simulink model "ctrl_student_HIL_Modules_withoutPathParam"  (R2015a)
settings: Solver=ode3  SolverMode=SingleTasking  StartTime=0.0  StopTime=inf  FixedStep=0.01  RelTol=1e-3
values from neighbouring files (symbols this model uses):
  D = [d_11 d_12 0 ... (first row only)    [ctrl_student_init.m]    (also in ctrl_student_observer_D.m = reshape([u.*(-3.545e-1)+u.^2.*3.787+6.555e-1,0.0,0.0,v.*2.44)
  eta_dot_ini = [7;0;0]    [Innput.m]    (also in Input_v3.m)
  K2 = diag([200,50,3])    [Input_v3.m]    (also in inputDPgains.m = [1 0 0; 0 1 0; 0 0 1])
  K_SZ = [1;1]    [Innput.m]
  l1 = [1 0 0;0 1 0;0 0 0.05]    [Input_v3.m]    (also in inputDPgains.m = [1 0 0; 0 1 0; 0 0 1])
  l2 = [1 0 0;0 1 0;0 0 0.05]    [Input_v3.m]    (also in inputDPgains.m = [1 0 0; 0 1 0; 0 0 1])
  l3 = [1 0 0;0 1 0;0 0 0.05]    [Input_v3.m]    (also in inputDPgains.m = [1 0 0; 0 1 0; 0 0 1])
  lim = [1.00;-20;6.45/2;-6.45/2]    [Innput.m]    (also in Input_v3.m = [20;-20;9;-9])
  lim_2 = [1.5;-22;7;-7]    [Innput.m]    (also in Input_v3.m = [25;-25;10;-10])
  M = [m_11 0    0 ... (first row only)    [ctrl_student_init.m]
libraries: dspstat3 x1, simulink x1
(part 1 of 3)
settings Model: CovSFcnEnable=off  Creator=mclab  LastModifiedBy=MCLab
settings OptimizationCC: BlockReduction=off  BooleanDataType=off
settings DebuggingCC: SaveWithParameterizedLinksMsg=none  UnderspecifiedInitializationDetection=Classic  MergeDetectMultiDrivingBlocksExec=none  SignalResolutionControl=TryResolveAllWithWarning
settings HardwareCC: TargetLongLongMode=on  TargetIntDivRoundTo=Zero  TargetEndianess=LittleEndian  TargetHWDeviceType=MATLAB Host  ProdEqTarget=off

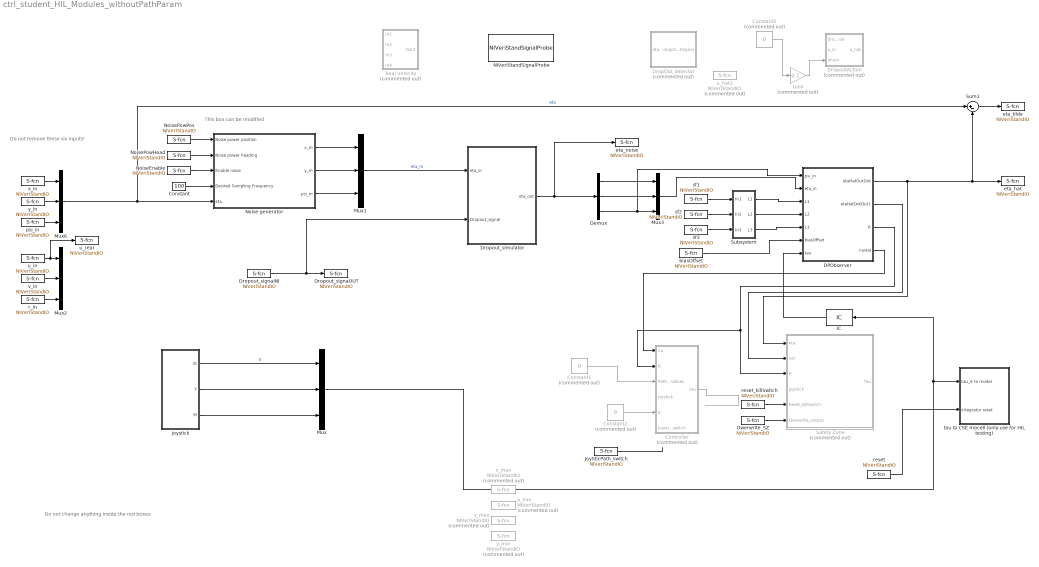
== system ctrl_student_HIL_Modules_withoutPathParam ==
  note: This box can be modified
  note: Do not change anything inside the red boxes
  note: Do not remove these six inputs!
  Constant : Constant  Value=100
  Constant1 : Constant  Commented=on  Value=0
  Constant2 : Constant  Commented=on  Value=0
  Constant5 : Constant  Commented=on  Value=0
  Controller : Subsystem  Commented=on
  DPObserver : Subsystem
  Demux : Demux  Outputs=3
  DropOut_detector : Subsystem  Commented=on
  DropoutAction : Subsystem  Commented=on
  Dropout_signaINl : S-Function  Priority=15  FunctionName=NIVeriStandIO  Parameters=width dtype portnum stime stype btype  mask(NI VeriStand Inport){portnum=15, width=-1, stime=-1, dtype=auto, stype=auto, btype=1}
      mask prompts: portnum "Port number:"; width "Port dimensions (-1 for dynamically sized):"; stime "Sample time (-1 for inherited):"; dtype "Data type:"; stype "Signal type:"; btype "Block type:"
      mask help: Use this inport on any level of nested subsystems to allow NI VeriStand software to map signals to it.
      mask init:
      | NIVeriStandIO_init;
      settings: CopyFcn=NIVeriStand_MDL_functions('', 'IO_copy');  DeleteFcn=NIVeriStand_MDL_functions('', 'IO_delete');  MoveFcn=set_param(gcb, 'Mask', 'on');
      mask Callback portnum: NIVeriStand_MDL_functions('', 'IO_setportnum');
      mask TypeOptions dtype: auto | double | single | int8 | uint8 | int16 | uint16 | int32 | uint32 | boolean
      mask Callback dtype: NIVeriStand_MDL_functions('', 'IO_booleansignal');
      mask TypeOptions stype: auto | real | complex
      mask Display:
      | patch([-x x], [-y y], [.90980 .81960 .32156]);
      | plot([xrad -x x xrad], [yrad -y y yrad]);
      | fprintf('NI In%d', portnum);
  Dropout_signaOUT : S-Function  Priority=5  FunctionName=NIVeriStandIO  Parameters=width dtype portnum stime stype btype  mask(NI VeriStand Outport){portnum=5, width=-1, stime=-1, dtype=auto, stype=auto, btype=0}
      mask prompts: portnum "Port number:"; width "Port dimensions (-1 for dynamically sized):"; stime "Sample time (-1 for inherited):"; dtype "Data type:"; stype "Signal type:"; btype "Block type:"
      mask help: Use this outport on any level of nested subsystems to allow NI VeriStand software to map signals to it.
      mask init:
      | NIVeriStandIO_init;
      settings: CopyFcn=NIVeriStand_MDL_functions('', 'IO_copy');  DeleteFcn=NIVeriStand_MDL_functions('', 'IO_delete');  MoveFcn=set_param(gcb, 'Mask', 'on');
      mask Callback portnum: NIVeriStand_MDL_functions('', 'IO_setportnum');
      mask TypeOptions dtype: auto | double | single | int8 | uint8 | int16 | uint16 | int32 | uint32 | boolean
      mask Callback dtype: NIVeriStand_MDL_functions('', 'IO_booleansignal');
      mask TypeOptions stype: auto | real | complex
      mask Display:
      | patch([-x x], [-y y], [.90980 .81960 .32156]);
      | plot([xrad -x x xrad], [yrad -y y yrad]);
      | fprintf('NI Out%d', portnum);
  Dropout_simulator : Subsystem
  Gain : Gain  Commented=on  Gain=0.1
  IC : InitialCondition  Value=[0;0;0]
  JoySticPath_switch : S-Function  Priority=16  FunctionName=NIVeriStandIO  Parameters=width dtype portnum stime stype btype  mask(NI VeriStand Inport){portnum=16, width=-1, stime=-1, dtype=auto, stype=auto, btype=1}
      mask prompts: portnum "Port number:"; width "Port dimensions (-1 for dynamically sized):"; stime "Sample time (-1 for inherited):"; dtype "Data type:"; stype "Signal type:"; btype "Block type:"
      mask help: Use this inport on any level of nested subsystems to allow NI VeriStand software to map signals to it.
      mask init:
      | NIVeriStandIO_init;
      settings: CopyFcn=NIVeriStand_MDL_functions('', 'IO_copy');  DeleteFcn=NIVeriStand_MDL_functions('', 'IO_delete');  MoveFcn=set_param(gcb, 'Mask', 'on');
      mask Callback portnum: NIVeriStand_MDL_functions('', 'IO_setportnum');
      mask TypeOptions dtype: auto | double | single | int8 | uint8 | int16 | uint16 | int32 | uint32 | boolean
      mask Callback dtype: NIVeriStand_MDL_functions('', 'IO_booleansignal');
      mask TypeOptions stype: auto | real | complex
      mask Display:
      | patch([-x x], [-y y], [.90980 .81960 .32156]);
      | plot([xrad -x x xrad], [yrad -y y yrad]);
      | fprintf('NI In%d', portnum);
  Mux{,1..3,6} (5 alike) : Mux  Inputs=3
  NIVeriStandSignalProbe : S-Function  FunctionName=NIVeriStandSignalProbe  Parameters=1
  Noise generator : Subsystem
  NoiseEnable : S-Function  Priority=5  FunctionName=NIVeriStandIO  Parameters=width dtype portnum stime stype btype  mask(NI VeriStand Inport){portnum=5, width=-1, stime=-1, dtype=auto, stype=auto, btype=1}
      mask prompts: portnum "Port number:"; width "Port dimensions (-1 for dynamically sized):"; stime "Sample time (-1 for inherited):"; dtype "Data type:"; stype "Signal type:"; btype "Block type:"
      mask help: Use this inport on any level of nested subsystems to allow NI VeriStand software to map signals to it.
      mask init:
      | NIVeriStandIO_init;
      settings: CopyFcn=NIVeriStand_MDL_functions('', 'IO_copy');  DeleteFcn=NIVeriStand_MDL_functions('', 'IO_delete');  MoveFcn=set_param(gcb, 'Mask', 'on');
      mask Callback portnum: NIVeriStand_MDL_functions('', 'IO_setportnum');
      mask TypeOptions dtype: auto | double | single | int8 | uint8 | int16 | uint16 | int32 | uint32 | boolean
      mask Callback dtype: NIVeriStand_MDL_functions('', 'IO_booleansignal');
      mask TypeOptions stype: auto | real | complex
      mask Display:
      | patch([-x x], [-y y], [.90980 .81960 .32156]);
      | plot([xrad -x x xrad], [yrad -y y yrad]);
      | fprintf('NI In%d', portnum);
  NoisePowHead : S-Function  Priority=6  FunctionName=NIVeriStandIO  Parameters=width dtype portnum stime stype btype  mask(NI VeriStand Inport){portnum=6, width=-1, stime=-1, dtype=auto, stype=auto, btype=1}
      mask prompts: portnum "Port number:"; width "Port dimensions (-1 for dynamically sized):"; stime "Sample time (-1 for inherited):"; dtype "Data type:"; stype "Signal type:"; btype "Block type:"
      mask help: Use this inport on any level of nested subsystems to allow NI VeriStand software to map signals to it.
      mask init:
      | NIVeriStandIO_init;
      settings: CopyFcn=NIVeriStand_MDL_functions('', 'IO_copy');  DeleteFcn=NIVeriStand_MDL_functions('', 'IO_delete');  MoveFcn=set_param(gcb, 'Mask', 'on');
      mask Callback portnum: NIVeriStand_MDL_functions('', 'IO_setportnum');
      mask TypeOptions dtype: auto | double | single | int8 | uint8 | int16 | uint16 | int32 | uint32 | boolean
      mask Callback dtype: NIVeriStand_MDL_functions('', 'IO_booleansignal');
      mask TypeOptions stype: auto | real | complex
      mask Display:
      | patch([-x x], [-y y], [.90980 .81960 .32156]);
      | plot([xrad -x x xrad], [yrad -y y yrad]);
      | fprintf('NI In%d', portnum);
  NoisePowPos : S-Function  Priority=9  FunctionName=NIVeriStandIO  Parameters=width dtype portnum stime stype btype  mask(NI VeriStand Inport){portnum=9, width=-1, stime=-1, dtype=auto, stype=auto, btype=1}
      mask prompts: portnum "Port number:"; width "Port dimensions (-1 for dynamically sized):"; stime "Sample time (-1 for inherited):"; dtype "Data type:"; stype "Signal type:"; btype "Block type:"
      mask help: Use this inport on any level of nested subsystems to allow NI VeriStand software to map signals to it.
      mask init:
      | NIVeriStandIO_init;
      settings: CopyFcn=NIVeriStand_MDL_functions('', 'IO_copy');  DeleteFcn=NIVeriStand_MDL_functions('', 'IO_delete');  MoveFcn=set_param(gcb, 'Mask', 'on');
      mask Callback portnum: NIVeriStand_MDL_functions('', 'IO_setportnum');
      mask TypeOptions dtype: auto | double | single | int8 | uint8 | int16 | uint16 | int32 | uint32 | boolean
      mask Callback dtype: NIVeriStand_MDL_functions('', 'IO_booleansignal');
      mask TypeOptions stype: auto | real | complex
      mask Display:
      | patch([-x x], [-y y], [.90980 .81960 .32156]);
      | plot([xrad -x x xrad], [yrad -y y yrad]);
      | fprintf('NI In%d', portnum);
  Owerwrite_SZ : S-Function  Priority=18  FunctionName=NIVeriStandIO  Parameters=width dtype portnum stime stype btype  mask(NI VeriStand Inport){portnum=18, width=-1, stime=-1, dtype=auto, stype=auto, btype=1}
      mask prompts: portnum "Port number:"; width "Port dimensions (-1 for dynamically sized):"; stime "Sample time (-1 for inherited):"; dtype "Data type:"; stype "Signal type:"; btype "Block type:"
      mask help: Use this inport on any level of nested subsystems to allow NI VeriStand software to map signals to it.
      mask init:
      | NIVeriStandIO_init;
      settings: CopyFcn=NIVeriStand_MDL_functions('', 'IO_copy');  DeleteFcn=NIVeriStand_MDL_functions('', 'IO_delete');  MoveFcn=set_param(gcb, 'Mask', 'on');
      mask Callback portnum: NIVeriStand_MDL_functions('', 'IO_setportnum');
      mask TypeOptions dtype: auto | double | single | int8 | uint8 | int16 | uint16 | int32 | uint32 | boolean
      mask Callback dtype: NIVeriStand_MDL_functions('', 'IO_booleansignal');
      mask TypeOptions stype: auto | real | complex
      mask Display:
      | patch([-x x], [-y y], [.90980 .81960 .32156]);
      | plot([xrad -x x xrad], [yrad -y y yrad]);
      | fprintf('NI In%d', portnum);
  Real Velocity : Subsystem  Commented=on
  "Safety Zone " : Subsystem  Commented=on
  Subsystem : Subsystem
  Sum1 : Sum  Inputs=|+-
  biasOffset : S-Function  Priority=13  FunctionName=NIVeriStandIO  Parameters=width dtype portnum stime stype btype  mask(NI VeriStand Inport){portnum=13, width=-1, stime=-1, dtype=auto, stype=auto, btype=1}
      mask prompts: portnum "Port number:"; width "Port dimensions (-1 for dynamically sized):"; stime "Sample time (-1 for inherited):"; dtype "Data type:"; stype "Signal type:"; btype "Block type:"
      mask help: Use this inport on any level of nested subsystems to allow NI VeriStand software to map signals to it.
      mask init:
      | NIVeriStandIO_init;
      settings: CopyFcn=NIVeriStand_MDL_functions('', 'IO_copy');  DeleteFcn=NIVeriStand_MDL_functions('', 'IO_delete');  MoveFcn=set_param(gcb, 'Mask', 'on');
      mask Callback portnum: NIVeriStand_MDL_functions('', 'IO_setportnum');
      mask TypeOptions dtype: auto | double | single | int8 | uint8 | int16 | uint16 | int32 | uint32 | boolean
      mask Callback dtype: NIVeriStand_MDL_functions('', 'IO_booleansignal');
      mask TypeOptions stype: auto | real | complex
      mask Display:
      | patch([-x x], [-y y], [.90980 .81960 .32156]);
      | plot([xrad -x x xrad], [yrad -y y yrad]);
      | fprintf('NI In%d', portnum);
  eta_hat : S-Function  Priority=1  FunctionName=NIVeriStandIO  Parameters=width dtype portnum stime stype btype  mask(NI VeriStand Outport){portnum=1, width=-1, stime=-1, dtype=auto, stype=auto, btype=0}
      mask prompts: portnum "Port number:"; width "Port dimensions (-1 for dynamically sized):"; stime "Sample time (-1 for inherited):"; dtype "Data type:"; stype "Signal type:"; btype "Block type:"
      mask help: Use this outport on any level of nested subsystems to allow NI VeriStand software to map signals to it.
      mask init:
      | NIVeriStandIO_init;
      settings: CopyFcn=NIVeriStand_MDL_functions('', 'IO_copy');  DeleteFcn=NIVeriStand_MDL_functions('', 'IO_delete');  MoveFcn=set_param(gcb, 'Mask', 'on');
      mask Callback portnum: NIVeriStand_MDL_functions('', 'IO_setportnum');
      mask TypeOptions dtype: auto | double | single | int8 | uint8 | int16 | uint16 | int32 | uint32 | boolean
      mask Callback dtype: NIVeriStand_MDL_functions('', 'IO_booleansignal');
      mask TypeOptions stype: auto | real | complex
      mask Display:
      | patch([-x x], [-y y], [.90980 .81960 .32156]);
      | plot([xrad -x x xrad], [yrad -y y yrad]);
      | fprintf('NI Out%d', portnum);
  eta_noise : S-Function  Priority=4  FunctionName=NIVeriStandIO  Parameters=width dtype portnum stime stype btype  mask(NI VeriStand Outport){portnum=4, width=-1, stime=-1, dtype=auto, stype=auto, btype=0}
      mask prompts: portnum "Port number:"; width "Port dimensions (-1 for dynamically sized):"; stime "Sample time (-1 for inherited):"; dtype "Data type:"; stype "Signal type:"; btype "Block type:"
      mask help: Use this outport on any level of nested subsystems to allow NI VeriStand software to map signals to it.
      mask init:
      | NIVeriStandIO_init;
      settings: CopyFcn=NIVeriStand_MDL_functions('', 'IO_copy');  DeleteFcn=NIVeriStand_MDL_functions('', 'IO_delete');  MoveFcn=set_param(gcb, 'Mask', 'on');
      mask Callback portnum: NIVeriStand_MDL_functions('', 'IO_setportnum');
      mask TypeOptions dtype: auto | double | single | int8 | uint8 | int16 | uint16 | int32 | uint32 | boolean
      mask Callback dtype: NIVeriStand_MDL_functions('', 'IO_booleansignal');
      mask TypeOptions stype: auto | real | complex
      mask Display:
      | patch([-x x], [-y y], [.90980 .81960 .32156]);
      | plot([xrad -x x xrad], [yrad -y y yrad]);
      | fprintf('NI Out%d', portnum);
  eta_tilde : S-Function  Priority=3  FunctionName=NIVeriStandIO  Parameters=width dtype portnum stime stype btype  mask(NI VeriStand Outport){portnum=3, width=-1, stime=-1, dtype=auto, stype=auto, btype=0}
      mask prompts: portnum "Port number:"; width "Port dimensions (-1 for dynamically sized):"; stime "Sample time (-1 for inherited):"; dtype "Data type:"; stype "Signal type:"; btype "Block type:"
      mask help: Use this outport on any level of nested subsystems to allow NI VeriStand software to map signals to it.
      mask init:
      | NIVeriStandIO_init;
      settings: CopyFcn=NIVeriStand_MDL_functions('', 'IO_copy');  DeleteFcn=NIVeriStand_MDL_functions('', 'IO_delete');  MoveFcn=set_param(gcb, 'Mask', 'on');
      mask Callback portnum: NIVeriStand_MDL_functions('', 'IO_setportnum');
      mask TypeOptions dtype: auto | double | single | int8 | uint8 | int16 | uint16 | int32 | uint32 | boolean
      mask Callback dtype: NIVeriStand_MDL_functions('', 'IO_booleansignal');
      mask TypeOptions stype: auto | real | complex
      mask Display:
      | patch([-x x], [-y y], [.90980 .81960 .32156]);
      | plot([xrad -x x xrad], [yrad -y y yrad]);
      | fprintf('NI Out%d', portnum);
  joystick : Subsystem
  psi_in : S-Function  Priority=2  FunctionName=NIVeriStandIO  Parameters=width dtype portnum stime stype btype  mask(NI VeriStand Inport){portnum=2, width=-1, stime=-1, dtype=auto, stype=auto, btype=1}
      mask prompts: portnum "Port number:"; width "Port dimensions (-1 for dynamically sized):"; stime "Sample time (-1 for inherited):"; dtype "Data type:"; stype "Signal type:"; btype "Block type:"
      mask help: Use this inport on any level of nested subsystems to allow NI VeriStand software to map signals to it.
      mask init:
      | NIVeriStandIO_init;
      settings: CopyFcn=NIVeriStand_MDL_functions('', 'IO_copy');  DeleteFcn=NIVeriStand_MDL_functions('', 'IO_delete');  MoveFcn=set_param(gcb, 'Mask', 'on');
      mask Callback portnum: NIVeriStand_MDL_functions('', 'IO_setportnum');
      mask TypeOptions dtype: auto | double | single | int8 | uint8 | int16 | uint16 | int32 | uint32 | boolean
      mask Callback dtype: NIVeriStand_MDL_functions('', 'IO_booleansignal');
      mask TypeOptions stype: auto | real | complex
      mask Display:
      | patch([-x x], [-y y], [.90980 .81960 .32156]);
      | plot([xrad -x x xrad], [yrad -y y yrad]);
      | fprintf('NI In%d', portnum);
  r_in : S-Function  Priority=4  FunctionName=NIVeriStandIO  Parameters=width dtype portnum stime stype btype  mask(NI VeriStand Inport){portnum=4, width=-1, stime=-1, dtype=auto, stype=auto, btype=1}
      mask prompts: portnum "Port number:"; width "Port dimensions (-1 for dynamically sized):"; stime "Sample time (-1 for inherited):"; dtype "Data type:"; stype "Signal type:"; btype "Block type:"
      mask help: Use this inport on any level of nested subsystems to allow NI VeriStand software to map signals to it.
      mask init:
      | NIVeriStandIO_init;
      settings: CopyFcn=NIVeriStand_MDL_functions('', 'IO_copy');  DeleteFcn=NIVeriStand_MDL_functions('', 'IO_delete');  MoveFcn=set_param(gcb, 'Mask', 'on');
      mask Callback portnum: NIVeriStand_MDL_functions('', 'IO_setportnum');
      mask TypeOptions dtype: auto | double | single | int8 | uint8 | int16 | uint16 | int32 | uint32 | boolean
      mask Callback dtype: NIVeriStand_MDL_functions('', 'IO_booleansignal');
      mask TypeOptions stype: auto | real | complex
      mask Display:
      | patch([-x x], [-y y], [.90980 .81960 .32156]);
      | plot([xrad -x x xrad], [yrad -y y yrad]);
      | fprintf('NI In%d', portnum);
  reset : S-Function  Priority=14  FunctionName=NIVeriStandIO  Parameters=width dtype portnum stime stype btype  mask(NI VeriStand Inport){portnum=14, width=-1, stime=-1, dtype=auto, stype=auto, btype=1}
      mask prompts: portnum "Port number:"; width "Port dimensions (-1 for dynamically sized):"; stime "Sample time (-1 for inherited):"; dtype "Data type:"; stype "Signal type:"; btype "Block type:"
      mask help: Use this inport on any level of nested subsystems to allow NI VeriStand software to map signals to it.
      mask init:
      | NIVeriStandIO_init;
      settings: CopyFcn=NIVeriStand_MDL_functions('', 'IO_copy');  DeleteFcn=NIVeriStand_MDL_functions('', 'IO_delete');  MoveFcn=set_param(gcb, 'Mask', 'on');
      mask Callback portnum: NIVeriStand_MDL_functions('', 'IO_setportnum');
      mask TypeOptions dtype: auto | double | single | int8 | uint8 | int16 | uint16 | int32 | uint32 | boolean
      mask Callback dtype: NIVeriStand_MDL_functions('', 'IO_booleansignal');
      mask TypeOptions stype: auto | real | complex
      mask Display:
      | patch([-x x], [-y y], [.90980 .81960 .32156]);
      | plot([xrad -x x xrad], [yrad -y y yrad]);
      | fprintf('NI In%d', portnum);
  reset_killSwitch : S-Function  Priority=17  FunctionName=NIVeriStandIO  Parameters=width dtype portnum stime stype btype  mask(NI VeriStand Inport){portnum=17, width=-1, stime=-1, dtype=auto, stype=auto, btype=1}
      mask prompts: portnum "Port number:"; width "Port dimensions (-1 for dynamically sized):"; stime "Sample time (-1 for inherited):"; dtype "Data type:"; stype "Signal type:"; btype "Block type:"
      mask help: Use this inport on any level of nested subsystems to allow NI VeriStand software to map signals to it.
      mask init:
      | NIVeriStandIO_init;
      settings: CopyFcn=NIVeriStand_MDL_functions('', 'IO_copy');  DeleteFcn=NIVeriStand_MDL_functions('', 'IO_delete');  MoveFcn=set_param(gcb, 'Mask', 'on');
      mask Callback portnum: NIVeriStand_MDL_functions('', 'IO_setportnum');
      mask TypeOptions dtype: auto | double | single | int8 | uint8 | int16 | uint16 | int32 | uint32 | boolean
      mask Callback dtype: NIVeriStand_MDL_functions('', 'IO_booleansignal');
      mask TypeOptions stype: auto | real | complex
      mask Display:
      | patch([-x x], [-y y], [.90980 .81960 .32156]);
      | plot([xrad -x x xrad], [yrad -y y yrad]);
      | fprintf('NI In%d', portnum);
  sf1 : S-Function  Priority=7  FunctionName=NIVeriStandIO  Parameters=width dtype portnum stime stype btype  mask(NI VeriStand Inport){portnum=7, width=-1, stime=-1, dtype=auto, stype=auto, btype=1}
      mask prompts: portnum "Port number:"; width "Port dimensions (-1 for dynamically sized):"; stime "Sample time (-1 for inherited):"; dtype "Data type:"; stype "Signal type:"; btype "Block type:"
      mask help: Use this inport on any level of nested subsystems to allow NI VeriStand software to map signals to it.
      mask init:
      | NIVeriStandIO_init;
      settings: CopyFcn=NIVeriStand_MDL_functions('', 'IO_copy');  DeleteFcn=NIVeriStand_MDL_functions('', 'IO_delete');  MoveFcn=set_param(gcb, 'Mask', 'on');
      mask Callback portnum: NIVeriStand_MDL_functions('', 'IO_setportnum');
      mask TypeOptions dtype: auto | double | single | int8 | uint8 | int16 | uint16 | int32 | uint32 | boolean
      mask Callback dtype: NIVeriStand_MDL_functions('', 'IO_booleansignal');
      mask TypeOptions stype: auto | real | complex
      mask Display:
      | patch([-x x], [-y y], [.90980 .81960 .32156]);
      | plot([xrad -x x xrad], [yrad -y y yrad]);
      | fprintf('NI In%d', portnum);
  sf2 : S-Function  Priority=11  FunctionName=NIVeriStandIO  Parameters=width dtype portnum stime stype btype  mask(NI VeriStand Inport){portnum=11, width=-1, stime=-1, dtype=auto, stype=auto, btype=1}
      mask prompts: portnum "Port number:"; width "Port dimensions (-1 for dynamically sized):"; stime "Sample time (-1 for inherited):"; dtype "Data type:"; stype "Signal type:"; btype "Block type:"
      mask help: Use this inport on any level of nested subsystems to allow NI VeriStand software to map signals to it.
      mask init:
      | NIVeriStandIO_init;
      settings: CopyFcn=NIVeriStand_MDL_functions('', 'IO_copy');  DeleteFcn=NIVeriStand_MDL_functions('', 'IO_delete');  MoveFcn=set_param(gcb, 'Mask', 'on');
      mask Callback portnum: NIVeriStand_MDL_functions('', 'IO_setportnum');
      mask TypeOptions dtype: auto | double | single | int8 | uint8 | int16 | uint16 | int32 | uint32 | boolean
      mask Callback dtype: NIVeriStand_MDL_functions('', 'IO_booleansignal');
      mask TypeOptions stype: auto | real | complex
      mask Display:
      | patch([-x x], [-y y], [.90980 .81960 .32156]);
      | plot([xrad -x x xrad], [yrad -y y yrad]);
      | fprintf('NI In%d', portnum);
  sf3 : S-Function  Priority=12  FunctionName=NIVeriStandIO  Parameters=width dtype portnum stime stype btype  mask(NI VeriStand Inport){portnum=12, width=-1, stime=-1, dtype=auto, stype=auto, btype=1}
      mask prompts: portnum "Port number:"; width "Port dimensions (-1 for dynamically sized):"; stime "Sample time (-1 for inherited):"; dtype "Data type:"; stype "Signal type:"; btype "Block type:"
      mask help: Use this inport on any level of nested subsystems to allow NI VeriStand software to map signals to it.
      mask init:
      | NIVeriStandIO_init;
      settings: CopyFcn=NIVeriStand_MDL_functions('', 'IO_copy');  DeleteFcn=NIVeriStand_MDL_functions('', 'IO_delete');  MoveFcn=set_param(gcb, 'Mask', 'on');
      mask Callback portnum: NIVeriStand_MDL_functions('', 'IO_setportnum');
      mask TypeOptions dtype: auto | double | single | int8 | uint8 | int16 | uint16 | int32 | uint32 | boolean
      mask Callback dtype: NIVeriStand_MDL_functions('', 'IO_booleansignal');
      mask TypeOptions stype: auto | real | complex
      mask Display:
      | patch([-x x], [-y y], [.90980 .81960 .32156]);
      | plot([xrad -x x xrad], [yrad -y y yrad]);
      | fprintf('NI In%d', portnum);
  tau to CSE mocell (only use for HIL testing) : Subsystem
  u_hat1 : S-Function  Priority=5  Commented=on  FunctionName=NIVeriStandIO  Parameters=width dtype portnum stime stype btype  mask(NI VeriStand Outport){portnum=5, width=-1, stime=-1, dtype=auto, stype=auto, btype=0}
      mask prompts: portnum "Port number:"; width "Port dimensions (-1 for dynamically sized):"; stime "Sample time (-1 for inherited):"; dtype "Data type:"; stype "Signal type:"; btype "Block type:"
      mask help: Use this outport on any level of nested subsystems to allow NI VeriStand software to map signals to it.
      mask init:
      | NIVeriStandIO_init;
      settings: CopyFcn=NIVeriStand_MDL_functions('', 'IO_copy');  DeleteFcn=NIVeriStand_MDL_functions('', 'IO_delete');  MoveFcn=set_param(gcb, 'Mask', 'on');
      mask Callback portnum: NIVeriStand_MDL_functions('', 'IO_setportnum');
      mask TypeOptions dtype: auto | double | single | int8 | uint8 | int16 | uint16 | int32 | uint32 | boolean
      mask Callback dtype: NIVeriStand_MDL_functions('', 'IO_booleansignal');
      mask TypeOptions stype: auto | real | complex
      mask Display:
      | patch([-x x], [-y y], [.90980 .81960 .32156]);
      | plot([xrad -x x xrad], [yrad -y y yrad]);
      | fprintf('NI Out%d', portnum);
  u_in : S-Function  Priority=10  FunctionName=NIVeriStandIO  Parameters=width dtype portnum stime stype btype  mask(NI VeriStand Inport){portnum=10, width=-1, stime=-1, dtype=auto, stype=auto, btype=1}
      mask prompts: portnum "Port number:"; width "Port dimensions (-1 for dynamically sized):"; stime "Sample time (-1 for inherited):"; dtype "Data type:"; stype "Signal type:"; btype "Block type:"
      mask help: Use this inport on any level of nested subsystems to allow NI VeriStand software to map signals to it.
      mask init:
      | NIVeriStandIO_init;
      settings: CopyFcn=NIVeriStand_MDL_functions('', 'IO_copy');  DeleteFcn=NIVeriStand_MDL_functions('', 'IO_delete');  MoveFcn=set_param(gcb, 'Mask', 'on');
      mask Callback portnum: NIVeriStand_MDL_functions('', 'IO_setportnum');
      mask TypeOptions dtype: auto | double | single | int8 | uint8 | int16 | uint16 | int32 | uint32 | boolean
      mask Callback dtype: NIVeriStand_MDL_functions('', 'IO_booleansignal');
      mask TypeOptions stype: auto | real | complex
      mask Display:
      | patch([-x x], [-y y], [.90980 .81960 .32156]);
      | plot([xrad -x x xrad], [yrad -y y yrad]);
      | fprintf('NI In%d', portnum);
  "u_real  " : S-Function  Priority=2  FunctionName=NIVeriStandIO  Parameters=width dtype portnum stime stype btype  mask(NI VeriStand Outport){portnum=2, width=-1, stime=-1, dtype=auto, stype=auto, btype=0}
      mask prompts: portnum "Port number:"; width "Port dimensions (-1 for dynamically sized):"; stime "Sample time (-1 for inherited):"; dtype "Data type:"; stype "Signal type:"; btype "Block type:"
      mask help: Use this outport on any level of nested subsystems to allow NI VeriStand software to map signals to it.
      mask init:
      | NIVeriStandIO_init;
      settings: CopyFcn=NIVeriStand_MDL_functions('', 'IO_copy');  DeleteFcn=NIVeriStand_MDL_functions('', 'IO_delete');  MoveFcn=set_param(gcb, 'Mask', 'on');
      mask Callback portnum: NIVeriStand_MDL_functions('', 'IO_setportnum');
      mask TypeOptions dtype: auto | double | single | int8 | uint8 | int16 | uint16 | int32 | uint32 | boolean
      mask Callback dtype: NIVeriStand_MDL_functions('', 'IO_booleansignal');
      mask TypeOptions stype: auto | real | complex
      mask Display:
      | patch([-x x], [-y y], [.90980 .81960 .32156]);
      | plot([xrad -x x xrad], [yrad -y y yrad]);
      | fprintf('NI Out%d', portnum);
  v_in : S-Function  Priority=8  FunctionName=NIVeriStandIO  Parameters=width dtype portnum stime stype btype  mask(NI VeriStand Inport){portnum=8, width=-1, stime=-1, dtype=auto, stype=auto, btype=1}
      mask prompts: portnum "Port number:"; width "Port dimensions (-1 for dynamically sized):"; stime "Sample time (-1 for inherited):"; dtype "Data type:"; stype "Signal type:"; btype "Block type:"
      mask help: Use this inport on any level of nested subsystems to allow NI VeriStand software to map signals to it.
      mask init:
      | NIVeriStandIO_init;
      settings: CopyFcn=NIVeriStand_MDL_functions('', 'IO_copy');  DeleteFcn=NIVeriStand_MDL_functions('', 'IO_delete');  MoveFcn=set_param(gcb, 'Mask', 'on');
      mask Callback portnum: NIVeriStand_MDL_functions('', 'IO_setportnum');
      mask TypeOptions dtype: auto | double | single | int8 | uint8 | int16 | uint16 | int32 | uint32 | boolean
      mask Callback dtype: NIVeriStand_MDL_functions('', 'IO_booleansignal');
      mask TypeOptions stype: auto | real | complex
      mask Display:
      | patch([-x x], [-y y], [.90980 .81960 .32156]);
      | plot([xrad -x x xrad], [yrad -y y yrad]);
      | fprintf('NI In%d', portnum);
  x_in : S-Function  Priority=3  FunctionName=NIVeriStandIO  Parameters=width dtype portnum stime stype btype  mask(NI VeriStand Inport){portnum=3, width=-1, stime=-1, dtype=auto, stype=auto, btype=1}
      mask prompts: portnum "Port number:"; width "Port dimensions (-1 for dynamically sized):"; stime "Sample time (-1 for inherited):"; dtype "Data type:"; stype "Signal type:"; btype "Block type:"
      mask help: Use this inport on any level of nested subsystems to allow NI VeriStand software to map signals to it.
      mask init:
      | NIVeriStandIO_init;
      settings: CopyFcn=NIVeriStand_MDL_functions('', 'IO_copy');  DeleteFcn=NIVeriStand_MDL_functions('', 'IO_delete');  MoveFcn=set_param(gcb, 'Mask', 'on');
      mask Callback portnum: NIVeriStand_MDL_functions('', 'IO_setportnum');
      mask TypeOptions dtype: auto | double | single | int8 | uint8 | int16 | uint16 | int32 | uint32 | boolean
      mask Callback dtype: NIVeriStand_MDL_functions('', 'IO_booleansignal');
      mask TypeOptions stype: auto | real | complex
      mask Display:
      | patch([-x x], [-y y], [.90980 .81960 .32156]);
      | plot([xrad -x x xrad], [yrad -y y yrad]);
      | fprintf('NI In%d', portnum);
  x_max : S-Function  Priority=16  Commented=on  FunctionName=NIVeriStandIO  Parameters=width dtype portnum stime stype btype  mask(NI VeriStand Inport){portnum=16, width=-1, stime=-1, dtype=auto, stype=auto, btype=1}
      mask prompts: portnum "Port number:"; width "Port dimensions (-1 for dynamically sized):"; stime "Sample time (-1 for inherited):"; dtype "Data type:"; stype "Signal type:"; btype "Block type:"
      mask help: Use this inport on any level of nested subsystems to allow NI VeriStand software to map signals to it.
      mask init:
      | NIVeriStandIO_init;
      settings: CopyFcn=NIVeriStand_MDL_functions('', 'IO_copy');  DeleteFcn=NIVeriStand_MDL_functions('', 'IO_delete');  MoveFcn=set_param(gcb, 'Mask', 'on');
      mask Callback portnum: NIVeriStand_MDL_functions('', 'IO_setportnum');
      mask TypeOptions dtype: auto | double | single | int8 | uint8 | int16 | uint16 | int32 | uint32 | boolean
      mask Callback dtype: NIVeriStand_MDL_functions('', 'IO_booleansignal');
      mask TypeOptions stype: auto | real | complex
      mask Display:
      | patch([-x x], [-y y], [.90980 .81960 .32156]);
      | plot([xrad -x x xrad], [yrad -y y yrad]);
      | fprintf('NI In%d', portnum);
  x_min : S-Function  Priority=7  Commented=on  FunctionName=NIVeriStandIO  Parameters=width dtype portnum stime stype btype  mask(NI VeriStand Inport){portnum=7, width=-1, stime=-1, dtype=auto, stype=auto, btype=1}
      mask prompts: portnum "Port number:"; width "Port dimensions (-1 for dynamically sized):"; stime "Sample time (-1 for inherited):"; dtype "Data type:"; stype "Signal type:"; btype "Block type:"
      mask help: Use this inport on any level of nested subsystems to allow NI VeriStand software to map signals to it.
      mask init:
      | NIVeriStandIO_init;
      settings: CopyFcn=NIVeriStand_MDL_functions('', 'IO_copy');  DeleteFcn=NIVeriStand_MDL_functions('', 'IO_delete');  MoveFcn=set_param(gcb, 'Mask', 'on');
      mask Callback portnum: NIVeriStand_MDL_functions('', 'IO_setportnum');
      mask TypeOptions dtype: auto | double | single | int8 | uint8 | int16 | uint16 | int32 | uint32 | boolean
      mask Callback dtype: NIVeriStand_MDL_functions('', 'IO_booleansignal');
      mask TypeOptions stype: auto | real | complex
      mask Display:
      | patch([-x x], [-y y], [.90980 .81960 .32156]);
      | plot([xrad -x x xrad], [yrad -y y yrad]);
      | fprintf('NI In%d', portnum);
  y_in : S-Function  Priority=1  FunctionName=NIVeriStandIO  Parameters=width dtype portnum stime stype btype  mask(NI VeriStand Inport){portnum=1, width=-1, stime=-1, dtype=auto, stype=auto, btype=1}
      mask prompts: portnum "Port number:"; width "Port dimensions (-1 for dynamically sized):"; stime "Sample time (-1 for inherited):"; dtype "Data type:"; stype "Signal type:"; btype "Block type:"
      mask help: Use this inport on any level of nested subsystems to allow NI VeriStand software to map signals to it.
      mask init:
      | NIVeriStandIO_init;
      settings: CopyFcn=NIVeriStand_MDL_functions('', 'IO_copy');  DeleteFcn=NIVeriStand_MDL_functions('', 'IO_delete');  MoveFcn=set_param(gcb, 'Mask', 'on');
      mask Callback portnum: NIVeriStand_MDL_functions('', 'IO_setportnum');
      mask TypeOptions dtype: auto | double | single | int8 | uint8 | int16 | uint16 | int32 | uint32 | boolean
      mask Callback dtype: NIVeriStand_MDL_functions('', 'IO_booleansignal');
      mask TypeOptions stype: auto | real | complex
      mask Display:
      | patch([-x x], [-y y], [.90980 .81960 .32156]);
      | plot([xrad -x x xrad], [yrad -y y yrad]);
      | fprintf('NI In%d', portnum);
  y_max : S-Function  Priority=9  Commented=on  FunctionName=NIVeriStandIO  Parameters=width dtype portnum stime stype btype  mask(NI VeriStand Inport){portnum=9, width=-1, stime=-1, dtype=auto, stype=auto, btype=1}
      mask prompts: portnum "Port number:"; width "Port dimensions (-1 for dynamically sized):"; stime "Sample time (-1 for inherited):"; dtype "Data type:"; stype "Signal type:"; btype "Block type:"
      mask help: Use this inport on any level of nested subsystems to allow NI VeriStand software to map signals to it.
      mask init:
      | NIVeriStandIO_init;
      settings: CopyFcn=NIVeriStand_MDL_functions('', 'IO_copy');  DeleteFcn=NIVeriStand_MDL_functions('', 'IO_delete');  MoveFcn=set_param(gcb, 'Mask', 'on');
      mask Callback portnum: NIVeriStand_MDL_functions('', 'IO_setportnum');
      mask TypeOptions dtype: auto | double | single | int8 | uint8 | int16 | uint16 | int32 | uint32 | boolean
      mask Callback dtype: NIVeriStand_MDL_functions('', 'IO_booleansignal');
      mask TypeOptions stype: auto | real | complex
      mask Display:
      | patch([-x x], [-y y], [.90980 .81960 .32156]);
      | plot([xrad -x x xrad], [yrad -y y yrad]);
      | fprintf('NI In%d', portnum);
  y_min : S-Function  Priority=10  Commented=on  FunctionName=NIVeriStandIO  Parameters=width dtype portnum stime stype btype  mask(NI VeriStand Inport){portnum=10, width=-1, stime=-1, dtype=auto, stype=auto, btype=1}
      mask prompts: portnum "Port number:"; width "Port dimensions (-1 for dynamically sized):"; stime "Sample time (-1 for inherited):"; dtype "Data type:"; stype "Signal type:"; btype "Block type:"
      mask help: Use this inport on any level of nested subsystems to allow NI VeriStand software to map signals to it.
      mask init:
      | NIVeriStandIO_init;
      settings: CopyFcn=NIVeriStand_MDL_functions('', 'IO_copy');  DeleteFcn=NIVeriStand_MDL_functions('', 'IO_delete');  MoveFcn=set_param(gcb, 'Mask', 'on');
      mask Callback portnum: NIVeriStand_MDL_functions('', 'IO_setportnum');
      mask TypeOptions dtype: auto | double | single | int8 | uint8 | int16 | uint16 | int32 | uint32 | boolean
      mask Callback dtype: NIVeriStand_MDL_functions('', 'IO_booleansignal');
      mask TypeOptions stype: auto | real | complex
      mask Display:
      | patch([-x x], [-y y], [.90980 .81960 .32156]);
      | plot([xrad -x x xrad], [yrad -y y yrad]);
      | fprintf('NI In%d', portnum);
  wires:
  x_in/1 -> Mux6/1
  y_in/1 -> Mux6/2
  psi_in/1 -> Mux6/3
  joystick/1(Xt) -> Mux/1  "X"
  u_in/1 -> "u_real  "/1, Mux2/1
  v_in/1 -> Mux2/2
  r_in/1 -> Mux2/3
  NoisePowHead/1 -> Noise generator/2(Noise power heading)
  NoisePowPos/1 -> Noise generator/1(Noise power position)
  NoiseEnable/1 -> Noise generator/3(Enable noise)
  Constant/1 -> Noise generator/4(Desired Sampling Frequency)
  Demux/3 -> Mux3/3, DPObserver/1(psi_in)
  Constant5/1 -> Gain/1
  Gain/1 -> DropoutAction/3(imuIn)
  Noise generator/1(x_m) -> Mux1/1
  Noise generator/2(y_m) -> Mux1/2
  Noise generator/3(psi_m) -> Mux1/3
  joystick/2(Y) -> Mux/2
  Mux6/1 -> Sum1/1, Noise generator/5(eta)  "eta"
  DPObserver/1(etaHatOutOut) -> "Safety Zone "/1(eta), eta_hat/1, Sum1/2
  Mux1/1 -> Dropout_simulator/1(eta_in)  "eta_m"
  joystick/3(M) -> Mux/3
  Demux/1 -> Mux3/1
  Demux/2 -> Mux3/2
  Mux3/1 -> DPObserver/2(eta_in)
  Sum1/1 -> eta_tilde/1
  biasOffset/1 -> DPObserver/6(biasOffset)
  reset/1 -> tau to CSE mocell (only use for HIL testing)/2(integrator reset)
  Dropout_signaINl/1 -> Dropout_signaOUT/1, Dropout_simulator/2(Dropout_signal)
  Dropout_simulator/1(eta_out) -> eta_noise/1, Demux/1
  sf1/1 -> Subsystem/1(In1)
  sf2/1 -> Subsystem/2(In2)
  sf3/1 -> Subsystem/3(In3)
  Subsystem/1(L1) -> DPObserver/3(L1)
  Subsystem/2(L2) -> DPObserver/4(L2)
  Subsystem/3(L3) -> DPObserver/5(L3)
  DPObserver/2(etaHatDotOut1) -> "Safety Zone "/2("vel ")
  DPObserver/3(R) -> Controller/2(R), "Safety Zone "/3(R)
  Controller/1(tau) -> ?
  DPObserver/4(nuHat) -> Controller/1(" nu")
  IC/1 -> DPObserver/7(tau)
  Constant1/1 -> Controller/3(Pathparametrization Values)
  Constant2/1 -> Controller/5(K)
  JoySticPath_switch/1 -> ?
  reset_killSwitch/1 -> "Safety Zone "/5(Reset_killSwitch)
  Owerwrite_SZ/1 -> "Safety Zone "/6(Overwrite_output)
  Mux/1 -> IC/1, tau to CSE mocell (only use for HIL testing)/1(tau_d to model)

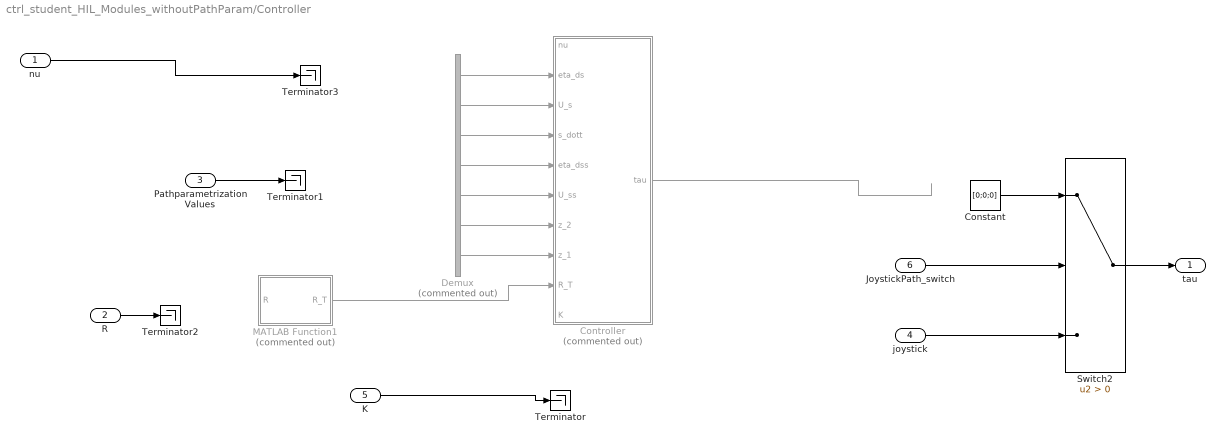
== system ctrl_student_HIL_Modules_withoutPathParam/Controller ==
  " nu" : Inport
  R : Inport  Port=2
  Pathparametrization Values : Inport  Port=3
  joystick : Inport  Port=4
  K : Inport  Port=5
  JoystickPath_switch : Inport  Port=6
  Constant : Constant  Value=[0;0;0]
  Controller : Subsystem  Commented=on
  Demux : Demux  Commented=on  Outputs=7
  MATLAB Function1 : MATLAB Function  Commented=on  TreatAsAtomicUnit=on
  Switch2 : Switch  Criteria=u2 > Threshold
  Terminator{,1..3} (4 alike) : Terminator
  tau : Outport
  wires:
  Pathparametrization Values/1 -> Terminator1/1
  Controller/1(tau) -> ?
  " nu"/1 -> Terminator3/1
  K/1 -> Terminator/1
  Switch2/1 -> tau/1
  joystick/1 -> Switch2/3
  JoystickPath_switch/1 -> Switch2/2
  MATLAB Function1/1(R_T) -> Controller/9(R_T)
  R/1 -> Terminator2/1
  Demux/1 -> Controller/2(eta_ds)
  Demux/2 -> Controller/3(U_s)
  Demux/3 -> Controller/4(s_dott)
  Demux/4 -> Controller/5(eta_dss)
  Demux/5 -> Controller/6(U_ss)
  Demux/6 -> Controller/7(z_2)
  Demux/7 -> Controller/8(z_1)
  Constant/1 -> Switch2/1

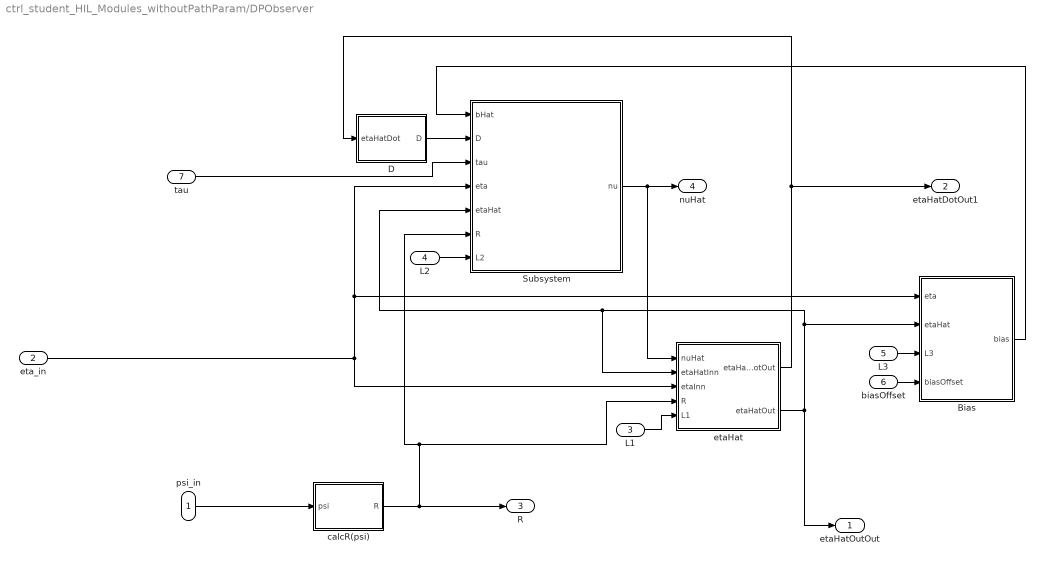
== system ctrl_student_HIL_Modules_withoutPathParam/DPObserver ==
  psi_in : Inport
  eta_in : Inport  Port=2
  L1 : Inport  Port=3
  L2 : Inport  Port=4
  L3 : Inport  Port=5
  biasOffset : Inport  Port=6
  tau : Inport  Port=7
  Bias : Subsystem
  D : MATLAB Function  TreatAsAtomicUnit=on
  Subsystem : Subsystem
  "calcR(psi) " : MATLAB Function  TreatAsAtomicUnit=on
  etaHat : Subsystem
  etaHatOutOut : Outport
  etaHatDotOut1 : Outport  Port=2
  R : Outport  Port=3
  nuHat : Outport  Port=4
  wires:
  "calcR(psi) "/1(R) -> R/1, Subsystem/6(R), etaHat/4(R)
  etaHat/2(etaHatOut) -> etaHatOutOut/1, Subsystem/5(etaHat), etaHat/2(etaHatInn), Bias/2(etaHat)
  tau/1 -> Subsystem/3(tau)
  etaHat/1(etaHatDotOut) -> etaHatDotOut1/1, D/1(etaHatDot)
  Subsystem/1(nu) -> nuHat/1, etaHat/1(nuHat)
  eta_in/1 -> etaHat/3(etaInn), Subsystem/4(eta), Bias/1(eta)
  D/1(D) -> Subsystem/2(D)
  Bias/1(bias) -> Subsystem/1(bHat)
  psi_in/1 -> "calcR(psi) "/1(psi)
  L2/1 -> Subsystem/7(L2)
  L1/1 -> etaHat/5(L1)
  L3/1 -> Bias/3(L3)
  biasOffset/1 -> Bias/4(biasOffset)

== system ctrl_student_HIL_Modules_withoutPathParam/DropOut_detector ==
  eta : Inport
  Display2 : Display  Commented=on
  Scope1 : Scope  Commented=on  NumInputPorts=2
      settings: ShowLegends=on  YMin=-0.22268~-5  YMax=0.33824~5
  Variance : dspstat3/Variance  Commented=on  run=off  reset_popup=None  directionMode=Each row  dimension=1  treatSBRowAsCol=off  roiEnable=off  roiType=Rectangles  roiPortion=Entire ROI  roiOutput=Individual statistics for each ROI  roiFlag=off  roundingMode=Floor  overflowMode=off
  dropoutDetect : MATLAB Function  TreatAsAtomicUnit=on
  etaHist Memory : DataStoreMemory  ReadBeforeWriteMsg=warning  WriteAfterWriteMsg=warning  WriteAfterReadMsg=warning  InitialValue=[0 1 2 3 4 5 6 7 8 9; 0 1 2 3 4 5 6 7 8 9; 0 1 2 3 4 5 6 7 8 9; 0 0 0 0 0 0 0 0 0 0]
  "etaHist_read " : DataStoreRead
  etaHist_write : DataStoreWrite
  dropOutSignal : Outport
  wires:
  "etaHist_read "/1 -> dropoutDetect/1(etaPrev)
  dropoutDetect/2(etaOut) -> Variance/1, etaHist_write/1
  Variance/1 -> Scope1/2, Display2/1
  dropoutDetect/1(dropout) -> dropOutSignal/1
  eta/1 -> dropoutDetect/2(eta)

== system ctrl_student_HIL_Modules_withoutPathParam/DropoutAction ==
  dropOutSignal : Inport
  u_in : Inport  Port=2
  imuIn : Inport  Port=3
  Integrator : Integrator
  Memory : Memory
  accInjection : MATLAB Function  TreatAsAtomicUnit=on
  u_hat : Outport
  wires:
  u_in/1 -> accInjection/3(uIn)
  Integrator/1 -> accInjection/4(dVel)
  Memory/1 -> accInjection/1(uLast)
  imuIn/1 -> Integrator/1
  accInjection/1(u_hat) -> Memory/1, u_hat/1
  dropOutSignal/1 -> accInjection/2(dropout)

== system ctrl_student_HIL_Modules_withoutPathParam/Dropout_simulator ==
  eta_in : Inport
  Dropout_signal : Inport  Port=2
  Demux : Demux  Outputs=3
  MATLAB Function : MATLAB Function  TreatAsAtomicUnit=on
  Memory : Memory
  Memory1 : Memory
  Memory2 : Memory
  Mux : Mux  Inputs=3
  eta_out : Outport
  wires:
  MATLAB Function/1(X_out) -> Mux/1, Memory2/1
  MATLAB Function/2(Y_out) -> Mux/2, Memory1/1
  MATLAB Function/3(Yaw_out) -> Mux/3, Memory/1
  Demux/2 -> MATLAB Function/2(Y_in)
  Demux/3 -> MATLAB Function/3(Yaw_in)
  Dropout_signal/1 -> MATLAB Function/4(Dropoutsignal)
  Memory/1 -> MATLAB Function/7(Yaw_prev)
  Memory1/1 -> MATLAB Function/6(Y_prev)
  Memory2/1 -> MATLAB Function/5(X_prev)
  Demux/1 -> MATLAB Function/1(X_in)
  eta_in/1 -> Demux/1
  Mux/1 -> eta_out/1

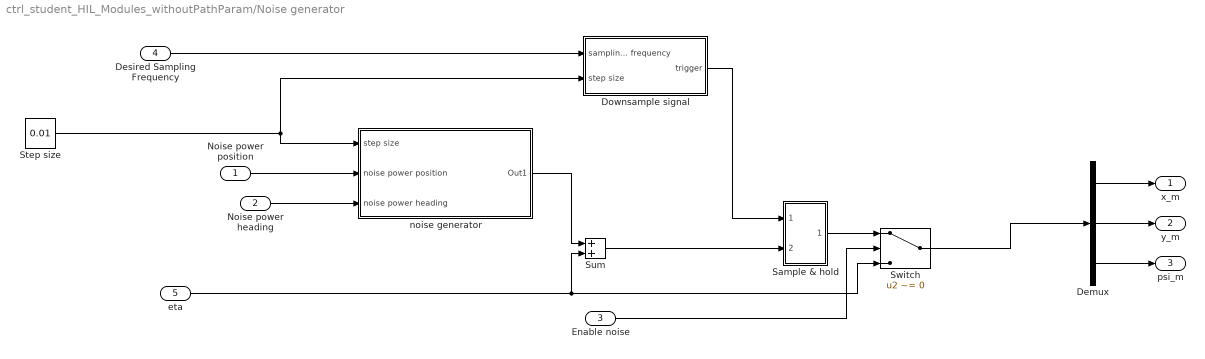
== system ctrl_student_HIL_Modules_withoutPathParam/Noise generator ==
  Noise power position : Inport
  Noise power heading : Inport  Port=2
  Enable noise : Inport  Port=3
  Desired Sampling Frequency : Inport  Port=4
  eta : Inport  Port=5
  Demux : Demux  Outputs=3
  Downsample	signal : Subsystem
  Sample & hold : Subsystem
  Step size : Constant  Value=0.01
  Sum : Sum
  Switch : Switch  Criteria=u2 ~= 0
  noise generator : Subsystem
  x_m : Outport
  y_m : Outport  Port=2
  psi_m : Outport  Port=3
  wires:
  Step size/1 -> Downsample	signal/2(step size), noise generator/1(step size)
  Downsample	signal/1(trigger) -> Sample & hold/1(trigger)
  Desired Sampling Frequency/1 -> Downsample	signal/1(sampling frequency)
  eta/1 -> Sum/2, Switch/3
  Sum/1 -> Sample & hold/2(input)
  Sample & hold/1(output) -> Switch/1
  Noise power position/1 -> noise generator/2(noise power position)
  Noise power heading/1 -> noise generator/3(noise power heading)
  noise generator/1(Out1) -> Sum/1
  Enable noise/1 -> Switch/2
  Switch/1 -> Demux/1
  Demux/3 -> psi_m/1
  Demux/2 -> y_m/1
  Demux/1 -> x_m/1

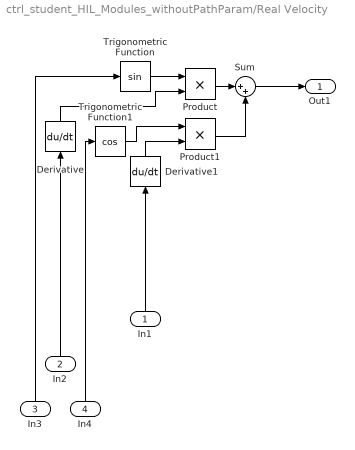
== system ctrl_student_HIL_Modules_withoutPathParam/Real Velocity ==
  In1 : Inport
  In2 : Inport  Port=2
  In3 : Inport  Port=3
  In4 : Inport  Port=4
  Derivative : Derivative
  Derivative1 : Derivative
  Product : Product
  Product1 : Product
  Sum : Sum  Inputs=|++
  Trigonometric Function : Trigonometry
  Trigonometric Function1 : Trigonometry  Operator=cos
  Out1 : Outport
  wires:
  Derivative/1 -> Product/2
  Trigonometric Function1/1 -> Product1/1
  Product/1 -> Sum/1
  Sum/1 -> Out1/1
  Trigonometric Function/1 -> Product/1
  Derivative1/1 -> Product1/2
  Product1/1 -> Sum/2
  In4/1 -> Trigonometric Function1/1
  In3/1 -> Trigonometric Function/1
  In1/1 -> Derivative1/1
  In2/1 -> Derivative/1

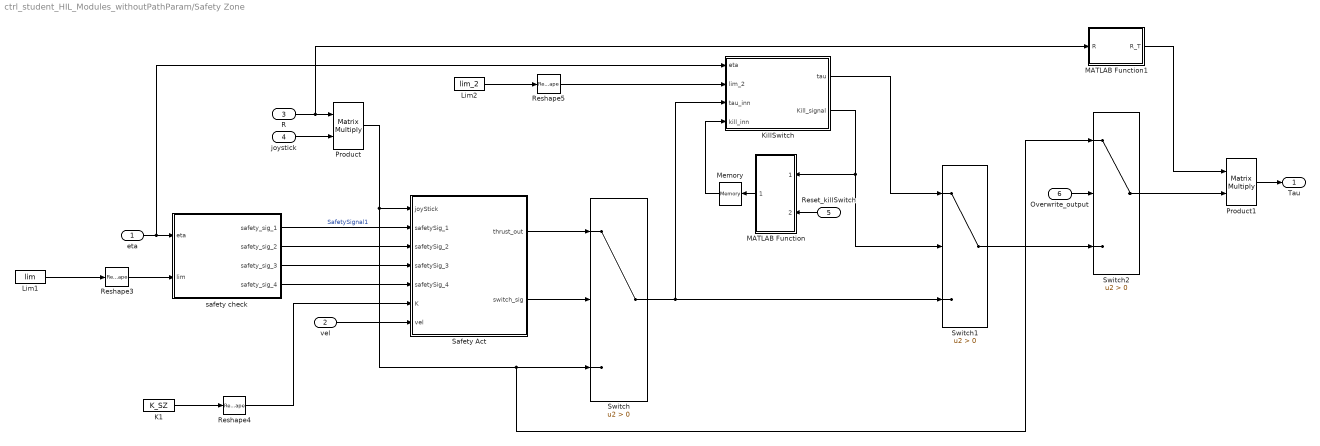
== system ctrl_student_HIL_Modules_withoutPathParam/Safety Zone  ==
  eta : Inport
  "vel " : Inport  Port=2
  R : Inport  Port=3
  joystick : Inport  Port=4
  Reset_killSwitch : Inport  Port=5
  Overwrite_output : Inport  Port=6
  K1 : Constant  Value=K_SZ
  KillSwitch : MATLAB Function  TreatAsAtomicUnit=on
  Lim1 : Constant  Value=lim
  Lim2 : Constant  Value=lim_2
  MATLAB Function : MATLAB Function  TreatAsAtomicUnit=on
  MATLAB Function1 : MATLAB Function  TreatAsAtomicUnit=on
  Memory : Memory
  Product : Product  Multiplication=Matrix(*)
  Product1 : Product  Multiplication=Matrix(*)
  Reshape3 : Reshape  OutputDimensionality=Customize  OutputDimensions=[4,1]
  Reshape4 : Reshape  OutputDimensionality=Customize  OutputDimensions=[2,1]
  Reshape5 : Reshape  OutputDimensionality=Customize  OutputDimensions=[4,1]
  Safety Act : MATLAB Function  TreatAsAtomicUnit=on
  Switch : Switch  Criteria=u2 > Threshold
  Switch1 : Switch  Criteria=u2 > Threshold
  Switch2 : Switch  Criteria=u2 > Threshold
  safety check : MATLAB Function  TreatAsAtomicUnit=on
  Tau : Outport
  wires:
  Product/1 -> Switch2/1, Switch/3, Safety Act/1(joyStick)
  safety check/1(safety_sig_1) -> Safety Act/2(safetySig_1)  "SafetySignal1"
  Safety Act/1(thrust_out) -> Switch/1
  safety check/2(safety_sig_2) -> Safety Act/3(safetySig_2)
  safety check/3(safety_sig_3) -> Safety Act/4(safetySig_3)
  safety check/4(safety_sig_4) -> Safety Act/5(safetySig_4)
  "vel "/1 -> Safety Act/7(vel)
  Reshape3/1 -> safety check/2(lim)
  Safety Act/2(switch_sig) -> Switch/2
  Reshape4/1 -> Safety Act/6(K)
  eta/1 -> KillSwitch/1(eta), safety check/1(eta)
  Reshape5/1 -> KillSwitch/2(lim_2)
  Memory/1 -> KillSwitch/4(kill_inn)
  Switch/1 -> KillSwitch/3(tau_inn), Switch1/3
  KillSwitch/1(tau) -> Switch1/1
  KillSwitch/2(Kill_signal) -> MATLAB Function/1(kill_signalInn), Switch1/2
  MATLAB Function/1(kill_signal) -> Memory/1
  Reset_killSwitch/1 -> MATLAB Function/2(Comand)
  Overwrite_output/1 -> Switch2/2
  Switch1/1 -> Switch2/3
  Switch2/1 -> Product1/2
  Lim1/1 -> Reshape3/1
  K1/1 -> Reshape4/1
  Lim2/1 -> Reshape5/1
  R/1 -> MATLAB Function1/1(R), Product/1
  joystick/1 -> Product/2
  MATLAB Function1/1(R_T) -> Product1/1
  Product1/1 -> Tau/1

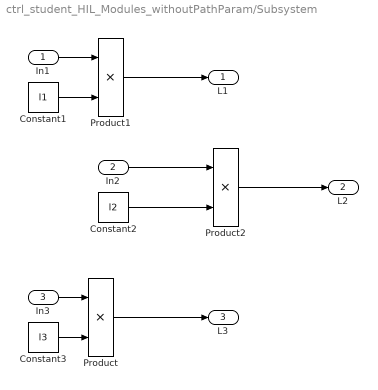
== system ctrl_student_HIL_Modules_withoutPathParam/Subsystem ==
  In1 : Inport
  In2 : Inport  Port=2
  In3 : Inport  Port=3
  Constant1 : Constant  Value=l1
  Constant2 : Constant  Value=l2
  Constant3 : Constant  Value=l3
  Product : Product
  Product1 : Product
  Product2 : Product
  L1 : Outport
  L2 : Outport  Port=2
  L3 : Outport  Port=3
  wires:
  Constant3/1 -> Product/2
  In1/1 -> Product1/1
  Constant2/1 -> Product2/2
  Product1/1 -> L1/1
  In2/1 -> Product2/1
  Product2/1 -> L2/1
  Constant1/1 -> Product1/2
  Product/1 -> L3/1
  In3/1 -> Product/1
